simulink library "MBDS_Subsystems"  (R2018b)
settings: Solver=ode45  StartTime=0.0  StopTime=10.0  RelTol=1e-3
undefined symbols (not defined in the file or in its folder): nbo_False, nbo_True
libraries: KIBES_Signal x1438, MBDS_Modules x44, simulink x2
(part 1 of 15)
Description:
  | MBDS project library for Subsystem models
settings Model: Creator=uid60719  LastModifiedBy=uie79669
settings DataIOCC: LimitDataPoints=on  SaveFormat=Array  SignalLoggingSaveFormat=ModelDataLogs
settings OptimizationCC: BlockReduction=off  BooleanDataType=off  ExpressionDepthLimit=2147483647  LifeSpan=inf
settings DebuggingCC: SaveWithParameterizedLinksMsg=none  UnderspecifiedInitializationDetection=Classic  MergeDetectMultiDrivingBlocksExec=none  SignalResolutionControl=TryResolveAllWithWarning  MultiTaskCondExecSysMsg=none  FcnCallInpInsideContextMsg=warning  AllowSymbolicDim=off  StateNameClashWarn=warning  SFUnexpectedBacktrackingDiag=warning  SFNoUnconditionalDefaultTransitionDiag=warning  SFExecutionAtInitializationDiag=none
settings HardwareCC: ProdBitPerPointer=32  ProdBitPerSizeT=32  ProdBitPerPtrDiffT=32  ProdLargestAtomicFloat=None  ProdIntDivRoundTo=Undefined  ProdEndianess=Unspecified  ProdWordSize=32  ProdHWDeviceType=32-bit Generic  TargetUnknown=on
settings ModelReferenceCC: PropagateSignalLabelsOutOfModel=off
settings SFSimCC: SimUseLocalCustomCode=off
settings RTWCC: RTWUseLocalCustomCode=off
settings CodeAppCC: StateflowObjectComments=on
settings GRTTargetCC: TargetLangStandard=C89/C90 (ANSI)  GeneratePreprocessorConditionals=Disable all  CombineOutputUpdateFcns=off  GRTInterface=on
settings ConfigComp: CovMetricSettings=dw  CovHtmlReporting=on  CovSaveCumulativeToWorkspaceVar=on  CovSaveSingleToWorkspaceVar=on  CovExternalEMLEnable=off  CovSFcnEnable=off

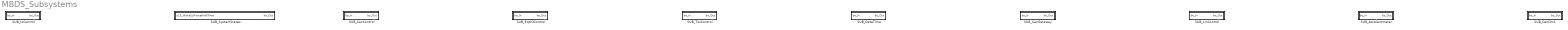
== system MBDS_Subsystems ==
  SUB_Accelerometer : Subsystem  Description=Controls accelerometer signals  mask(SUB_Accelerometer){MBDS_ElementType=Subsystem, MBDS_WorkStatus=In Work, MBDS_LastModified=2023-02-23-17:58:48}
      mask prompts: MBDS_ElementType "MBDS element type:"; MBDS_WorkStatus "Work status:"; MBDS_LastModified "Last modified:"
      mask help: Controls accelerometer signals
      mask Help: eval(['open([workdir(''help_dir:''),''\MBDS_ProjectLibrary.html''])'])
      mask Display: disp('V 1.3')
  SUB_CanControl : Subsystem  Description=CAN Control  mask(SUB_CanControl){MBDS_ElementType=Subsystem, MBDS_WorkStatus=In Work, MBDS_LastModified=2023-02-23-17:58:52}
      mask prompts: MBDS_ElementType "MBDS element type:"; MBDS_WorkStatus "Work status:"; MBDS_LastModified "Last modified:"
      mask help: CAN Control
      mask Help: eval(['open([workdir(''help_dir:''),''\MBDS_ProjectLibrary.html''])'])
      mask Display: disp('V 1.16')
  SUB_CanDm1 : Subsystem  Description=Check DM1 Rx/Tx  mask(SUB_CanDm1){MBDS_ElementType=Subsystem, MBDS_WorkStatus=In Work, MBDS_LastModified=2023-02-23-17:58:48}
      mask prompts: MBDS_ElementType "MBDS element type:"; MBDS_WorkStatus "Work status:"; MBDS_LastModified "Last modified:"
      mask help: Check DM1 Rx/Tx
      mask Help: eval(['open([workdir(''help_dir:''),''\MBDS_ProjectLibrary.html''])'])
      mask Display: disp('V 1.11')
  SUB_CanGateway : Subsystem  Description=CAN Gateways.  mask(SUB_CanGateway){MBDS_ElementType=Subsystem, MBDS_WorkStatus=In Work, MBDS_LastModified=2023-02-23-17:58:50}
      mask prompts: MBDS_ElementType "MBDS element type:"; MBDS_WorkStatus "Work status:"; MBDS_LastModified "Last modified:"
      mask help: CAN Gateways.
      mask Help: eval(['open([workdir(''help_dir:''),''\MBDS_ProjectLibrary.html''])'])
      mask Display: disp('V 1.6')
  SUB_DateTime : Subsystem  Description=Date and Time Control  mask(SUB_DateTime){MBDS_ElementType=Subsystem, MBDS_WorkStatus=In Work, MBDS_LastModified=2023-02-23-17:58:50}
      mask prompts: MBDS_ElementType "MBDS element type:"; MBDS_WorkStatus "Work status:"; MBDS_LastModified "Last modified:"
      mask help: Date and Time Control
      mask Help: eval(['open([workdir(''help_dir:''),''\MBDS_ProjectLibrary.html''])'])
      mask Display: disp('V 1.7')
  SUB_ExpIOControl : Subsystem  Description=Expansion Input/Output Control  mask(SUB_ExpIOControl){MBDS_ElementType=Subsystem, MBDS_WorkStatus=In Work, MBDS_LastModified=2023-02-23-17:58:54}
      mask prompts: MBDS_ElementType "MBDS element type:"; MBDS_WorkStatus "Work status:"; MBDS_LastModified "Last modified:"
      mask help: Expansion Input/Output Control
      mask Help: eval(['open([workdir(''help_dir:''),''\MBDS_ProjectLibrary.html''])'])
      mask Display: disp('V 1.101')
  SUB_IoControl : Subsystem  Description=Input/Output Control  mask(SUB_IoControl){MBDS_ElementType=Subsystem, MBDS_WorkStatus=In Work, MBDS_LastModified=2023-02-23-17:58:58}
      mask prompts: MBDS_ElementType "MBDS element type:"; MBDS_WorkStatus "Work status:"; MBDS_LastModified "Last modified:"
      mask help: Input/Output Control
      mask Help: eval(['open([workdir(''help_dir:''),''\MBDS_ProjectLibrary.html''])'])
      mask Display: disp('V 1.107')
  SUB_LinControl : Subsystem  Description=LIN Control  mask(SUB_LinControl){MBDS_ElementType=Subsystem, MBDS_WorkStatus=In Work, MBDS_LastModified=2023-02-23-17:58:49}
      mask prompts: MBDS_ElementType "MBDS element type:"; MBDS_WorkStatus "Work status:"; MBDS_LastModified "Last modified:"
      mask help: LIN Control
      mask Help: eval(['open([workdir(''help_dir:''),''\MBDS_ProjectLibrary.html''])'])
      mask Display: disp('V 1.27')
  SUB_SystemStates : Subsystem  Description=System States  mask(SUB_SystemStates){MBDS_ElementType=Subsystem, MBDS_WorkStatus=In Work, MBDS_LastModified=2023-02-23-17:58:59}
      mask prompts: MBDS_ElementType "MBDS element type:"; MBDS_WorkStatus "Work status:"; MBDS_LastModified "Last modified:"
      mask help: System States
      mask Help: eval(['open([workdir(''help_dir:''),''\MBDS_ProjectLibrary.html''])'])
      mask Display: disp('V 1.17')
  SUB_TsuControl : Subsystem  Description=TSU Control  mask(SUB_TsuControl){MBDS_ElementType=Subsystem, MBDS_WorkStatus=In Work, MBDS_LastModified=2023-02-23-17:58:51}
      mask prompts: MBDS_ElementType "MBDS element type:"; MBDS_WorkStatus "Work status:"; MBDS_LastModified "Last modified:"
      mask help: TSU Control
      mask Help: eval(['open([workdir(''help_dir:''),''\MBDS_ProjectLibrary.html''])'])
      mask Display: disp('V 1.4')

== system MBDS_Subsystems/SUB_Accelerometer ==
  bo_In : Inport  OutDataTypeStr=boolean
  Constant : Constant  InitFcn=|  Value=true  OutDataTypeStr=boolean
      | if(exist('MBDS_BlockCallback', 'file'))
      |    MBDS_BlockCallback('Update', gcb);  
      | end
  Data Type Conversion : DataTypeConversion  InitFcn=|
      | try
      |    MBDS_BlockCallback('Update', gcb);
      | end
      settings: AttributesFormatString=Saturate: %<SaturateOnIntegerOverflow>
  Data Type Conversion1 : DataTypeConversion  InitFcn=|
      | try
      |    MBDS_BlockCallback('Update', gcb);
      | end
      settings: AttributesFormatString=Saturate: %<SaturateOnIntegerOverflow>
  Data Type Conversion2 : DataTypeConversion  InitFcn=|
      | try
      |    MBDS_BlockCallback('Update', gcb);
      | end
      settings: AttributesFormatString=Saturate: %<SaturateOnIntegerOverflow>
  Ground : Ground  InitFcn=|
      | try
      |    MBDS_BlockCallback('Update', gcb);
      | end
      settings: MoveFcn=UpdateBlockSize(gcb);
  Terminator : Terminator
      settings: MoveFcn=UpdateBlockSize(gcb);
      settings: InitFcn=|
      | try
      |    MBDS_BlockCallback('Update', gcb);
      | end
  in_INOUT_RAMDevice.boSystemWake : KIBES_Signal/KIBES_Signal  MBDS_LibraryBlock=on  DatabaseKey=3  SignalName=INOUT_RAMDevice.boSystemWake  SymbolName=INOUT_RAMDevice_boSystemWake_000003  DataType=boolean  Init=0  Slope=1  Bias=0  DataSize=1  fpDataType=boolean  BlockIOType=Inport  DeviceType=0
  in_IN_InertianSensor.Accelerometer.Ax : KIBES_Signal/KIBES_Signal  MBDS_LibraryBlock=on  DatabaseKey=2138  SignalName=IN_InertianSensor.Accelerometer.Ax  SymbolName=IN_InertianSensor_Accelerometer_Ax_002138  DataType=int16  Init=0  Slope=1  Bias=0  DataSize=1  fpDataType=int16  BlockIOType=Inport  DeviceType=0
  in_IN_InertianSensor.Accelerometer.Ay : KIBES_Signal/KIBES_Signal  MBDS_LibraryBlock=on  DatabaseKey=2137  SignalName=IN_InertianSensor.Accelerometer.Ay  SymbolName=IN_InertianSensor_Accelerometer_Ay_002137  DataType=int16  Init=0  Slope=1  Bias=0  DataSize=1  fpDataType=int16  BlockIOType=Inport  DeviceType=0
  in_IN_InertianSensor.Accelerometer.Az : KIBES_Signal/KIBES_Signal  MBDS_LibraryBlock=on  DatabaseKey=2136  SignalName=IN_InertianSensor.Accelerometer.Az  SymbolName=IN_InertianSensor_Accelerometer_Az_002136  DataType=int16  Init=0  Slope=1  Bias=0  DataSize=1  fpDataType=int16  BlockIOType=Inport  DeviceType=0
  out_OUT_InertianSensor.Accelerometer.DeviceEnable : KIBES_Signal/KIBES_Signal  MBDS_LibraryBlock=on  DatabaseKey=2135  SignalName=OUT_InertianSensor.Accelerometer.DeviceEnable  SymbolName=OUT_InertianSensor_Accelerometer_DeviceEnable_002135  DataType=boolean  Init=0  Slope=1  Bias=0  DataSize=1  fpDataType=boolean  BlockIOType=Outport  DeviceType=0
  out_OUT_PCAN.Tx_Acc.ACCELEROMETER.MessageEnable : KIBES_Signal/KIBES_Signal  MBDS_LibraryBlock=on  DatabaseKey=2134  SignalName=OUT_PCAN.Tx_Acc.ACCELEROMETER.MessageEnable  SymbolName=OUT_PCAN_Tx_Acc_ACCELEROMETER_MessageEnable_002134  DataType=boolean  Init=0  Slope=1  Bias=0  DataSize=1  fpDataType=boolean  BlockIOType=Outport  DeviceType=0
  out_OUT_PCAN.Tx_Acc.ACCELEROMETER.X : KIBES_Signal/KIBES_Signal  MBDS_LibraryBlock=on  DatabaseKey=2131  SignalName=OUT_PCAN.Tx_Acc.ACCELEROMETER.X  SymbolName=OUT_PCAN_Tx_Acc_ACCELEROMETER_X_002131  DataType=uint16  Init=0  Slope=1  Bias=0  DataSize=1  fpDataType=uint16  BlockIOType=Outport  DeviceType=0
  out_OUT_PCAN.Tx_Acc.ACCELEROMETER.Y : KIBES_Signal/KIBES_Signal  MBDS_LibraryBlock=on  DatabaseKey=2132  SignalName=OUT_PCAN.Tx_Acc.ACCELEROMETER.Y  SymbolName=OUT_PCAN_Tx_Acc_ACCELEROMETER_Y_002132  DataType=uint16  Init=0  Slope=1  Bias=0  DataSize=1  fpDataType=uint16  BlockIOType=Outport  DeviceType=0
  out_OUT_PCAN.Tx_Acc.ACCELEROMETER.Z : KIBES_Signal/KIBES_Signal  MBDS_LibraryBlock=on  DatabaseKey=2133  SignalName=OUT_PCAN.Tx_Acc.ACCELEROMETER.Z  SymbolName=OUT_PCAN_Tx_Acc_ACCELEROMETER_Z_002133  DataType=uint16  Init=0  Slope=1  Bias=0  DataSize=1  fpDataType=uint16  BlockIOType=Outport  DeviceType=0
  bo_Out : Outport  OutDataTypeStr=boolean
  wires:
  Data Type Conversion2/1 -> out_OUT_PCAN.Tx_Acc.ACCELEROMETER.Z/1
  Data Type Conversion1/1 -> out_OUT_PCAN.Tx_Acc.ACCELEROMETER.Y/1
  Data Type Conversion/1 -> out_OUT_PCAN.Tx_Acc.ACCELEROMETER.X/1
  in_IN_InertianSensor.Accelerometer.Az/1 -> Data Type Conversion2/1
  in_IN_InertianSensor.Accelerometer.Ay/1 -> Data Type Conversion1/1
  in_IN_InertianSensor.Accelerometer.Ax/1 -> Data Type Conversion/1
  Constant/1 -> out_OUT_InertianSensor.Accelerometer.DeviceEnable/1
  in_INOUT_RAMDevice.boSystemWake/1 -> out_OUT_PCAN.Tx_Acc.ACCELEROMETER.MessageEnable/1
  Ground/1 -> bo_Out/1  "bo_Out"
  bo_In/1 -> Terminator/1

== system MBDS_Subsystems/SUB_CanControl ==
  note: Enable Message Forwarding
  note: SleepMode(0)
      | ShutdownMode(1)
      | ASWFailureMode(2)
      | ModeOverVoltage(3)
      | ModeUnderVoltage(4)
      | LCWakeupSequence(5)
      | TimeoutFailureMode(6)
      |  ActiveMode(7)
      |  SYFlashingMode(8)
  bo_In : Inport  OutDataTypeStr=boolean
  Constant : Constant  InitFcn=|  Value=true  OutDataTypeStr=boolean
      | if(exist('MBDS_BlockCallback', 'file'))
      |    MBDS_BlockCallback('Update', gcb);  
      | end
  Ground : Ground  InitFcn=|
      | try
      |    MBDS_BlockCallback('Update', gcb);
      | end
      settings: MoveFcn=UpdateBlockSize(gcb);
  Terminator : Terminator
      settings: MoveFcn=UpdateBlockSize(gcb);
      settings: InitFcn=|
      | try
      |    MBDS_BlockCallback('Update', gcb);
      | end
  WakeUpSequency : Stateflow chart  TreatAsAtomicUnit=on
      settings: CopyFcn=|
      | if(exist('MBDS_BlockCallback', 'file'))
      |    MBDS_BlockCallback('Copy', gcb);
      | end
  in_IN_DigitalInputs.IN_DIG_36 : KIBES_Signal/KIBES_Signal  MBDS_LibraryBlock=on  DatabaseKey=60  SignalName=IN_DigitalInputs.IN_DIG_36  SymbolName=IN_DigitalInputs_IN_DIG_36_000060  DataType=boolean  Init=0  Slope=1  Bias=0  DataSize=1  fpDataType=boolean  BlockIOType=Inport  DeviceType=0
  out_OUT_ACAN.MessageForwardingEnable : KIBES_Signal/KIBES_Signal  MBDS_LibraryBlock=on  DatabaseKey=2356  SignalName=OUT_ACAN.MessageForwardingEnable  SymbolName=OUT_ACAN_MessageForwardingEnable_002356  DataType=boolean  Init=0  Slope=1  Bias=0  DataSize=1  fpDataType=boolean  BlockIOType=Outport  DeviceType=0
  out_OUT_DCAN.MessageForwardingEnable : KIBES_Signal/KIBES_Signal  MBDS_LibraryBlock=on  DatabaseKey=1337  SignalName=OUT_DCAN.MessageForwardingEnable  SymbolName=OUT_DCAN_MessageForwardingEnable_001337  DataType=boolean  Init=0  Slope=1  Bias=0  DataSize=1  fpDataType=boolean  BlockIOType=Outport  DeviceType=0
  out_OUT_DRCAN.MessageForwardingEnable : KIBES_Signal/KIBES_Signal  MBDS_LibraryBlock=on  DatabaseKey=1335  SignalName=OUT_DRCAN.MessageForwardingEnable  SymbolName=OUT_DRCAN_MessageForwardingEnable_001335  DataType=boolean  Init=0  Slope=1  Bias=0  DataSize=1  fpDataType=boolean  BlockIOType=Outport  DeviceType=0
  out_OUT_FMSCAN.MessageForwardingEnable : KIBES_Signal/KIBES_Signal  MBDS_LibraryBlock=on  DatabaseKey=1336  SignalName=OUT_FMSCAN.MessageForwardingEnable  SymbolName=OUT_FMSCAN_MessageForwardingEnable_001336  DataType=boolean  Init=0  Slope=1  Bias=0  DataSize=1  fpDataType=boolean  BlockIOType=Outport  DeviceType=0
  out_OUT_HCAN.MessageForwardingEnable : KIBES_Signal/KIBES_Signal  MBDS_LibraryBlock=on  DatabaseKey=1340  SignalName=OUT_HCAN.MessageForwardingEnable  SymbolName=OUT_HCAN_MessageForwardingEnable_001340  DataType=boolean  Init=0  Slope=1  Bias=0  DataSize=1  fpDataType=boolean  BlockIOType=Outport  DeviceType=0
  out_OUT_ICAN.BSG_TX_18DA1721.Ctrl50_FcnDA1.MessageEnable : KIBES_Signal/KIBES_Signal  MBDS_LibraryBlock=on  DatabaseKey=2793  SignalName=OUT_ICAN.BSG_TX_18DA1721.Ctrl50_FcnDA1.MessageEnable  SymbolName=OUT_ICAN_BSG_TX_18DA1721_Ctrl50_FcnDA1_MessageEnable_002793  DataType=boolean  Init=0  Slope=1  Bias=0  DataSize=1  fpDataType=boolean  BlockIOType=Outport  DeviceType=0
  out_OUT_ICAN.BSG_TX_18DA1721.Ctrl50_FcnDA2.MessageEnable : KIBES_Signal/KIBES_Signal  MBDS_LibraryBlock=on  DatabaseKey=2795  SignalName=OUT_ICAN.BSG_TX_18DA1721.Ctrl50_FcnDA2.MessageEnable  SymbolName=OUT_ICAN_BSG_TX_18DA1721_Ctrl50_FcnDA2_MessageEnable_002795  DataType=boolean  Init=0  Slope=1  Bias=0  DataSize=1  fpDataType=boolean  BlockIOType=Outport  DeviceType=0
  out_OUT_ICAN.BSG_TX_18DA1721.Ctrl50_ScrDA1.MessageEnable : KIBES_Signal/KIBES_Signal  MBDS_LibraryBlock=on  DatabaseKey=2796  SignalName=OUT_ICAN.BSG_TX_18DA1721.Ctrl50_ScrDA1.MessageEnable  SymbolName=OUT_ICAN_BSG_TX_18DA1721_Ctrl50_ScrDA1_MessageEnable_002796  DataType=boolean  Init=0  Slope=1  Bias=0  DataSize=1  fpDataType=boolean  BlockIOType=Outport  DeviceType=0
  out_OUT_ICAN.BSG_TX_18DA1721.Ctrl50_ScrDA2.MessageEnable : KIBES_Signal/KIBES_Signal  MBDS_LibraryBlock=on  DatabaseKey=2797  SignalName=OUT_ICAN.BSG_TX_18DA1721.Ctrl50_ScrDA2.MessageEnable  SymbolName=OUT_ICAN_BSG_TX_18DA1721_Ctrl50_ScrDA2_MessageEnable_002797  DataType=boolean  Init=0  Slope=1  Bias=0  DataSize=1  fpDataType=boolean  BlockIOType=Outport  DeviceType=0
  out_OUT_ICAN.BSG_TX_18DA1721.Ctrl50_SubView.MessageEnable : KIBES_Signal/KIBES_Signal  MBDS_LibraryBlock=on  DatabaseKey=2794  SignalName=OUT_ICAN.BSG_TX_18DA1721.Ctrl50_SubView.MessageEnable  SymbolName=OUT_ICAN_BSG_TX_18DA1721_Ctrl50_SubView_MessageEnable_002794  DataType=boolean  Init=0  Slope=1  Bias=0  DataSize=1  fpDataType=boolean  BlockIOType=Outport  DeviceType=0
  out_OUT_ICAN.BSG_TX_18DA1721.ICHMI1CTRL.MessageEnable : KIBES_Signal/KIBES_Signal  MBDS_LibraryBlock=on  DatabaseKey=2798  SignalName=OUT_ICAN.BSG_TX_18DA1721.ICHMI1CTRL.MessageEnable  SymbolName=OUT_ICAN_BSG_TX_18DA1721_ICHMI1CTRL_MessageEnable_002798  DataType=boolean  Init=0  Slope=1  Bias=0  DataSize=1  fpDataType=boolean  BlockIOType=Outport  DeviceType=0
  out_OUT_ICAN.BSG_TX_18DA1721.ICOM1CTRL.ICOMCtrl : KIBES_Signal/KIBES_Signal  MBDS_LibraryBlock=on  DatabaseKey=2704  SignalName=OUT_ICAN.BSG_TX_18DA1721.ICOM1CTRL.ICOMCtrl  SymbolName=OUT_ICAN_BSG_TX_18DA1721_ICOM1CTRL_ICOMCtrl_002704  DataType=uint8  Init=1  Slope=1  Bias=0  DataSize=1  fpDataType=uint8  BlockIOType=Outport  DeviceType=0
  out_OUT_ICAN.BSG_TX_18DA1721.ICOM1CTRL.MessageEnable : KIBES_Signal/KIBES_Signal  MBDS_LibraryBlock=on  DatabaseKey=2792  SignalName=OUT_ICAN.BSG_TX_18DA1721.ICOM1CTRL.MessageEnable  SymbolName=OUT_ICAN_BSG_TX_18DA1721_ICOM1CTRL_MessageEnable_002792  DataType=boolean  Init=0  Slope=1  Bias=0  DataSize=1  fpDataType=boolean  BlockIOType=Outport  DeviceType=0
  out_OUT_ICAN.MessageForwardingEnable : KIBES_Signal/KIBES_Signal  MBDS_LibraryBlock=on  DatabaseKey=1342  SignalName=OUT_ICAN.MessageForwardingEnable  SymbolName=OUT_ICAN_MessageForwardingEnable_001342  DataType=boolean  Init=0  Slope=1  Bias=0  DataSize=1  fpDataType=boolean  BlockIOType=Outport  DeviceType=0
  out_OUT_PCAN.MessageForwardingEnable : KIBES_Signal/KIBES_Signal  MBDS_LibraryBlock=on  DatabaseKey=1347  SignalName=OUT_PCAN.MessageForwardingEnable  SymbolName=OUT_PCAN_MessageForwardingEnable_001347  DataType=boolean  Init=0  Slope=1  Bias=0  DataSize=1  fpDataType=boolean  BlockIOType=Outport  DeviceType=0
  bo_Out : Outport  OutDataTypeStr=boolean
  wires:
  in_IN_DigitalInputs.IN_DIG_36/1 -> WakeUpSequency/1(bo_TRM15)
  WakeUpSequency/1(u8_IControlsts) -> out_OUT_ICAN.BSG_TX_18DA1721.ICOM1CTRL.ICOMCtrl/1
  Constant/1 -> out_OUT_DCAN.MessageForwardingEnable/1, out_OUT_DRCAN.MessageForwardingEnable/1, out_OUT_FMSCAN.MessageForwardingEnable/1, out_OUT_HCAN.MessageForwardingEnable/1, out_OUT_ICAN.MessageForwardingEnable/1, out_OUT_PCAN.MessageForwardingEnable/1, out_OUT_ACAN.MessageForwardingEnable/1, out_OUT_ICAN.BSG_TX_18DA1721.Ctrl50_ScrDA2.MessageEnable/1, out_OUT_ICAN.BSG_TX_18DA1721.Ctrl50_FcnDA1.MessageEnable/1, out_OUT_ICAN.BSG_TX_18DA1721.Ctrl50_FcnDA2.MessageEnable/1, out_OUT_ICAN.BSG_TX_18DA1721.Ctrl50_ScrDA1.MessageEnable/1, out_OUT_ICAN.BSG_TX_18DA1721.Ctrl50_SubView.MessageEnable/1, out_OUT_ICAN.BSG_TX_18DA1721.ICHMI1CTRL.MessageEnable/1, out_OUT_ICAN.BSG_TX_18DA1721.ICOM1CTRL.MessageEnable/1
  Ground/1 -> bo_Out/1  "bo_Out"
  bo_In/1 -> Terminator/1

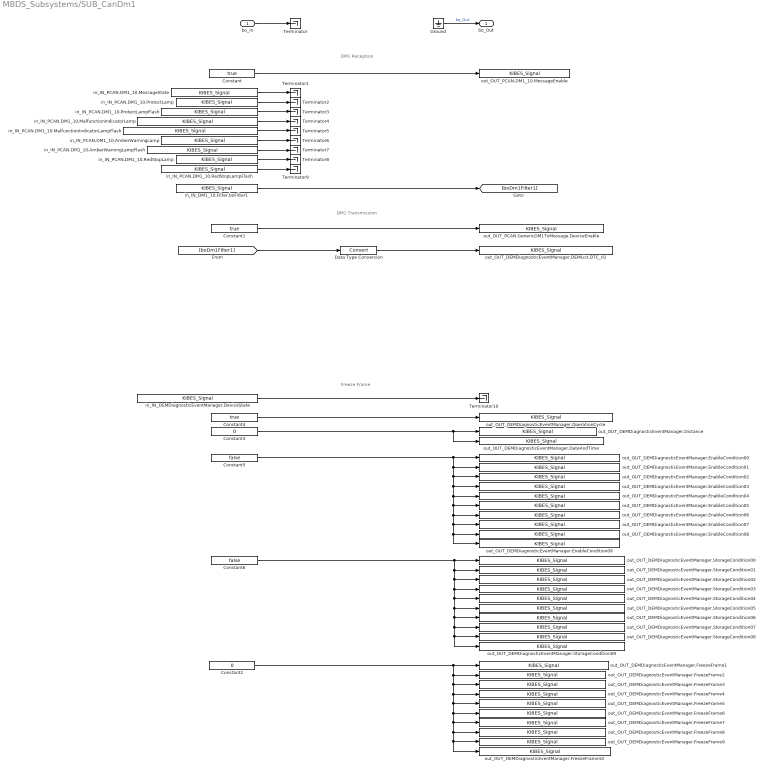
== system MBDS_Subsystems/SUB_CanDm1 ==
  note: Freeze Frame
  note: DM1 Transmission
  note: DM1 Reception
  bo_In : Inport  OutDataTypeStr=boolean
  Constant : Constant  InitFcn=|  Value=true  OutDataTypeStr=boolean
      | if(exist('MBDS_BlockCallback', 'file'))
      |    MBDS_BlockCallback('Update', gcb);  
      | end
  Constant1 : Constant  InitFcn=|  Value=true  OutDataTypeStr=boolean
      | if(exist('MBDS_BlockCallback', 'file'))
      |    MBDS_BlockCallback('Update', gcb);  
      | end
  Constant2 : Constant  InitFcn=|  Value=0  OutDataTypeStr=uint16
      | if(exist('MBDS_BlockCallback', 'file'))
      |    MBDS_BlockCallback('Update', gcb);  
      | end
  Constant3 : Constant  InitFcn=|  Value=0  OutDataTypeStr=uint32
      | if(exist('MBDS_BlockCallback', 'file'))
      |    MBDS_BlockCallback('Update', gcb);  
      | end
  Constant4 : Constant  InitFcn=|  Value=true  OutDataTypeStr=boolean
      | if(exist('MBDS_BlockCallback', 'file'))
      |    MBDS_BlockCallback('Update', gcb);  
      | end
  Constant5 : Constant  InitFcn=|  Value=false  OutDataTypeStr=boolean
      | if(exist('MBDS_BlockCallback', 'file'))
      |    MBDS_BlockCallback('Update', gcb);  
      | end
  Constant6 : Constant  InitFcn=|  Value=false  OutDataTypeStr=boolean
      | if(exist('MBDS_BlockCallback', 'file'))
      |    MBDS_BlockCallback('Update', gcb);  
      | end
  Data Type Conversion : DataTypeConversion  InitFcn=|
      | try
      |    MBDS_BlockCallback('Update', gcb);
      | end
      settings: AttributesFormatString=Saturate: %<SaturateOnIntegerOverflow>
  Ground : Ground  InitFcn=|
      | try
      |    MBDS_BlockCallback('Update', gcb);
      | end
      settings: MoveFcn=UpdateBlockSize(gcb);
  Terminator{,1..10} (11 alike) : Terminator
      settings: MoveFcn=UpdateBlockSize(gcb);
      settings: InitFcn=|
      | try
      |    MBDS_BlockCallback('Update', gcb);
      | end
  in_IN_DEMDiagnosticEventManager.DeviceState : KIBES_Signal/KIBES_Signal  MBDS_LibraryBlock=on  DatabaseKey=2238  SignalName=IN_DEMDiagnosticEventManager.DeviceState  SymbolName=IN_DEMDiagnosticEventManager_DeviceState_002238  DataType=uint16  Init=0  Slope=1  Bias=0  DataSize=1  fpDataType=uint16  BlockIOType=Inport  DeviceType=0
  in_IN_DM1_10.Filter.boFilter1 : KIBES_Signal/KIBES_Signal  MBDS_LibraryBlock=on  DatabaseKey=2234  SignalName=IN_DM1_10.Filter.boFilter1  SymbolName=IN_DM1_10_Filter_boFilter1_002234  DataType=boolean  Init=0  Slope=1  Bias=0  DataSize=1  fpDataType=boolean  BlockIOType=Inport  DeviceType=0
  in_IN_PCAN.DM1_10.AmberWarningLamp : KIBES_Signal/KIBES_Signal  MBDS_LibraryBlock=on  DatabaseKey=2233  SignalName=IN_PCAN.DM1_10.AmberWarningLamp  SymbolName=IN_PCAN_DM1_10_AmberWarningLamp_002233  DataType=boolean  Init=0  Slope=1  Bias=0  DataSize=1  fpDataType=boolean  BlockIOType=Inport  DeviceType=0
  in_IN_PCAN.DM1_10.AmberWarningLampFlash : KIBES_Signal/KIBES_Signal  MBDS_LibraryBlock=on  DatabaseKey=2232  SignalName=IN_PCAN.DM1_10.AmberWarningLampFlash  SymbolName=IN_PCAN_DM1_10_AmberWarningLampFlash_002232  DataType=uint8  Init=0  Slope=1  Bias=0  DataSize=1  fpDataType=uint8  BlockIOType=Inport  DeviceType=0
  in_IN_PCAN.DM1_10.MalfunctionIndicatorLamp : KIBES_Signal/KIBES_Signal  MBDS_LibraryBlock=on  DatabaseKey=2231  SignalName=IN_PCAN.DM1_10.MalfunctionIndicatorLamp  SymbolName=IN_PCAN_DM1_10_MalfunctionIndicatorLamp_002231  DataType=boolean  Init=0  Slope=1  Bias=0  DataSize=1  fpDataType=boolean  BlockIOType=Inport  DeviceType=0
  in_IN_PCAN.DM1_10.MalfunctionIndicatorLampFlash : KIBES_Signal/KIBES_Signal  MBDS_LibraryBlock=on  DatabaseKey=2230  SignalName=IN_PCAN.DM1_10.MalfunctionIndicatorLampFlash  SymbolName=IN_PCAN_DM1_10_MalfunctionIndicatorLampFlash_002230  DataType=uint8  Init=0  Slope=1  Bias=0  DataSize=1  fpDataType=uint8  BlockIOType=Inport  DeviceType=0
  in_IN_PCAN.DM1_10.MessageState : KIBES_Signal/KIBES_Signal  MBDS_LibraryBlock=on  DatabaseKey=2228  SignalName=IN_PCAN.DM1_10.MessageState  SymbolName=IN_PCAN_DM1_10_MessageState_002228  DataType=uint16  Init=0  Slope=1  Bias=0  DataSize=1  fpDataType=uint16  BlockIOType=Inport  DeviceType=0
  in_IN_PCAN.DM1_10.ProtectLamp : KIBES_Signal/KIBES_Signal  MBDS_LibraryBlock=on  DatabaseKey=2227  SignalName=IN_PCAN.DM1_10.ProtectLamp  SymbolName=IN_PCAN_DM1_10_ProtectLamp_002227  DataType=boolean  Init=0  Slope=1  Bias=0  DataSize=1  fpDataType=boolean  BlockIOType=Inport  DeviceType=0
  in_IN_PCAN.DM1_10.ProtectLampFlash : KIBES_Signal/KIBES_Signal  MBDS_LibraryBlock=on  DatabaseKey=2226  SignalName=IN_PCAN.DM1_10.ProtectLampFlash  SymbolName=IN_PCAN_DM1_10_ProtectLampFlash_002226  DataType=uint8  Init=0  Slope=1  Bias=0  DataSize=1  fpDataType=uint8  BlockIOType=Inport  DeviceType=0
  in_IN_PCAN.DM1_10.RedStopLamp : KIBES_Signal/KIBES_Signal  MBDS_LibraryBlock=on  DatabaseKey=2225  SignalName=IN_PCAN.DM1_10.RedStopLamp  SymbolName=IN_PCAN_DM1_10_RedStopLamp_002225  DataType=boolean  Init=0  Slope=1  Bias=0  DataSize=1  fpDataType=boolean  BlockIOType=Inport  DeviceType=0
  in_IN_PCAN.DM1_10.RedStopLampFlash : KIBES_Signal/KIBES_Signal  MBDS_LibraryBlock=on  DatabaseKey=2224  SignalName=IN_PCAN.DM1_10.RedStopLampFlash  SymbolName=IN_PCAN_DM1_10_RedStopLampFlash_002224  DataType=uint8  Init=0  Slope=1  Bias=0  DataSize=1  fpDataType=uint8  BlockIOType=Inport  DeviceType=0
  out_OUT_DEMDiagnosticEventManager.DEMList.DTC_01 : KIBES_Signal/KIBES_Signal  MBDS_LibraryBlock=on  DatabaseKey=2237  SignalName=OUT_DEMDiagnosticEventManager.DEMList.DTC_01  SymbolName=OUT_DEMDiagnosticEventManager_DEMList_DTC_01_002237  DataType=uint8  Init=0  Slope=1  Bias=0  DataSize=1  fpDataType=uint8  BlockIOType=Outport  DeviceType=0
  out_OUT_DEMDiagnosticEventManager.DateAndTime : KIBES_Signal/KIBES_Signal  MBDS_LibraryBlock=on  DatabaseKey=2242  SignalName=OUT_DEMDiagnosticEventManager.DateAndTime  SymbolName=OUT_DEMDiagnosticEventManager_DateAndTime_002242  DataType=uint32  Init=0  Slope=1  Bias=0  DataSize=1  fpDataType=uint32  BlockIOType=Outport  DeviceType=0
  out_OUT_DEMDiagnosticEventManager.Distance : KIBES_Signal/KIBES_Signal  MBDS_LibraryBlock=on  DatabaseKey=2243  SignalName=OUT_DEMDiagnosticEventManager.Distance  SymbolName=OUT_DEMDiagnosticEventManager_Distance_002243  DataType=uint32  Init=0  Slope=1  Bias=0  DataSize=1  fpDataType=uint32  BlockIOType=Outport  DeviceType=0
  out_OUT_DEMDiagnosticEventManager.EnableCondition00 : KIBES_Signal/KIBES_Signal  MBDS_LibraryBlock=on  DatabaseKey=2239  SignalName=OUT_DEMDiagnosticEventManager.EnableCondition00  SymbolName=OUT_DEMDiagnosticEventManager_EnableCondition00_002239  DataType=boolean  Init=0  Slope=1  Bias=0  DataSize=1  fpDataType=boolean  BlockIOType=Outport  DeviceType=0
  out_OUT_DEMDiagnosticEventManager.EnableCondition01 : KIBES_Signal/KIBES_Signal  MBDS_LibraryBlock=on  DatabaseKey=2245  SignalName=OUT_DEMDiagnosticEventManager.EnableCondition01  SymbolName=OUT_DEMDiagnosticEventManager_EnableCondition01_002245  DataType=boolean  Init=0  Slope=1  Bias=0  DataSize=1  fpDataType=boolean  BlockIOType=Outport  DeviceType=0
  out_OUT_DEMDiagnosticEventManager.EnableCondition02 : KIBES_Signal/KIBES_Signal  MBDS_LibraryBlock=on  DatabaseKey=2246  SignalName=OUT_DEMDiagnosticEventManager.EnableCondition02  SymbolName=OUT_DEMDiagnosticEventManager_EnableCondition02_002246  DataType=boolean  Init=0  Slope=1  Bias=0  DataSize=1  fpDataType=boolean  BlockIOType=Outport  DeviceType=0
  out_OUT_DEMDiagnosticEventManager.EnableCondition03 : KIBES_Signal/KIBES_Signal  MBDS_LibraryBlock=on  DatabaseKey=2247  SignalName=OUT_DEMDiagnosticEventManager.EnableCondition03  SymbolName=OUT_DEMDiagnosticEventManager_EnableCondition03_002247  DataType=boolean  Init=0  Slope=1  Bias=0  DataSize=1  fpDataType=boolean  BlockIOType=Outport  DeviceType=0
  out_OUT_DEMDiagnosticEventManager.EnableCondition04 : KIBES_Signal/KIBES_Signal  MBDS_LibraryBlock=on  DatabaseKey=2248  SignalName=OUT_DEMDiagnosticEventManager.EnableCondition04  SymbolName=OUT_DEMDiagnosticEventManager_EnableCondition04_002248  DataType=boolean  Init=0  Slope=1  Bias=0  DataSize=1  fpDataType=boolean  BlockIOType=Outport  DeviceType=0
  out_OUT_DEMDiagnosticEventManager.EnableCondition05 : KIBES_Signal/KIBES_Signal  MBDS_LibraryBlock=on  DatabaseKey=2249  SignalName=OUT_DEMDiagnosticEventManager.EnableCondition05  SymbolName=OUT_DEMDiagnosticEventManager_EnableCondition05_002249  DataType=boolean  Init=0  Slope=1  Bias=0  DataSize=1  fpDataType=boolean  BlockIOType=Outport  DeviceType=0
  out_OUT_DEMDiagnosticEventManager.EnableCondition06 : KIBES_Signal/KIBES_Signal  MBDS_LibraryBlock=on  DatabaseKey=2250  SignalName=OUT_DEMDiagnosticEventManager.EnableCondition06  SymbolName=OUT_DEMDiagnosticEventManager_EnableCondition06_002250  DataType=boolean  Init=0  Slope=1  Bias=0  DataSize=1  fpDataType=boolean  BlockIOType=Outport  DeviceType=0
  out_OUT_DEMDiagnosticEventManager.EnableCondition07 : KIBES_Signal/KIBES_Signal  MBDS_LibraryBlock=on  DatabaseKey=2251  SignalName=OUT_DEMDiagnosticEventManager.EnableCondition07  SymbolName=OUT_DEMDiagnosticEventManager_EnableCondition07_002251  DataType=boolean  Init=0  Slope=1  Bias=0  DataSize=1  fpDataType=boolean  BlockIOType=Outport  DeviceType=0
  out_OUT_DEMDiagnosticEventManager.EnableCondition08 : KIBES_Signal/KIBES_Signal  MBDS_LibraryBlock=on  DatabaseKey=2252  SignalName=OUT_DEMDiagnosticEventManager.EnableCondition08  SymbolName=OUT_DEMDiagnosticEventManager_EnableCondition08_002252  DataType=boolean  Init=0  Slope=1  Bias=0  DataSize=1  fpDataType=boolean  BlockIOType=Outport  DeviceType=0
  out_OUT_DEMDiagnosticEventManager.EnableCondition09 : KIBES_Signal/KIBES_Signal  MBDS_LibraryBlock=on  DatabaseKey=2244  SignalName=OUT_DEMDiagnosticEventManager.EnableCondition09  SymbolName=OUT_DEMDiagnosticEventManager_EnableCondition09_002244  DataType=boolean  Init=0  Slope=1  Bias=0  DataSize=1  fpDataType=boolean  BlockIOType=Outport  DeviceType=0
  out_OUT_DEMDiagnosticEventManager.FreezeFrame1 : KIBES_Signal/KIBES_Signal  MBDS_LibraryBlock=on  DatabaseKey=2241  SignalName=OUT_DEMDiagnosticEventManager.FreezeFrame1  SymbolName=OUT_DEMDiagnosticEventManager_FreezeFrame1_002241  DataType=uint16  Init=0  Slope=1  Bias=0  DataSize=1  fpDataType=uint16  BlockIOType=Outport  DeviceType=0
  out_OUT_DEMDiagnosticEventManager.FreezeFrame10 : KIBES_Signal/KIBES_Signal  MBDS_LibraryBlock=on  DatabaseKey=2270  SignalName=OUT_DEMDiagnosticEventManager.FreezeFrame10  SymbolName=OUT_DEMDiagnosticEventManager_FreezeFrame10_002270  DataType=uint16  Init=0  Slope=1  Bias=0  DataSize=1  fpDataType=uint16  BlockIOType=Outport  DeviceType=0
  out_OUT_DEMDiagnosticEventManager.FreezeFrame2 : KIBES_Signal/KIBES_Signal  MBDS_LibraryBlock=on  DatabaseKey=2253  SignalName=OUT_DEMDiagnosticEventManager.FreezeFrame2  SymbolName=OUT_DEMDiagnosticEventManager_FreezeFrame2_002253  DataType=uint16  Init=0  Slope=1  Bias=0  DataSize=1  fpDataType=uint16  BlockIOType=Outport  DeviceType=0
  out_OUT_DEMDiagnosticEventManager.FreezeFrame3 : KIBES_Signal/KIBES_Signal  MBDS_LibraryBlock=on  DatabaseKey=2254  SignalName=OUT_DEMDiagnosticEventManager.FreezeFrame3  SymbolName=OUT_DEMDiagnosticEventManager_FreezeFrame3_002254  DataType=uint16  Init=0  Slope=1  Bias=0  DataSize=1  fpDataType=uint16  BlockIOType=Outport  DeviceType=0
  out_OUT_DEMDiagnosticEventManager.FreezeFrame4 : KIBES_Signal/KIBES_Signal  MBDS_LibraryBlock=on  DatabaseKey=2255  SignalName=OUT_DEMDiagnosticEventManager.FreezeFrame4  SymbolName=OUT_DEMDiagnosticEventManager_FreezeFrame4_002255  DataType=uint16  Init=0  Slope=1  Bias=0  DataSize=1  fpDataType=uint16  BlockIOType=Outport  DeviceType=0
  out_OUT_DEMDiagnosticEventManager.FreezeFrame5 : KIBES_Signal/KIBES_Signal  MBDS_LibraryBlock=on  DatabaseKey=2256  SignalName=OUT_DEMDiagnosticEventManager.FreezeFrame5  SymbolName=OUT_DEMDiagnosticEventManager_FreezeFrame5_002256  DataType=uint16  Init=0  Slope=1  Bias=0  DataSize=1  fpDataType=uint16  BlockIOType=Outport  DeviceType=0
  out_OUT_DEMDiagnosticEventManager.FreezeFrame6 : KIBES_Signal/KIBES_Signal  MBDS_LibraryBlock=on  DatabaseKey=2266  SignalName=OUT_DEMDiagnosticEventManager.FreezeFrame6  SymbolName=OUT_DEMDiagnosticEventManager_FreezeFrame6_002266  DataType=uint16  Init=0  Slope=1  Bias=0  DataSize=1  fpDataType=uint16  BlockIOType=Outport  DeviceType=0
  out_OUT_DEMDiagnosticEventManager.FreezeFrame7 : KIBES_Signal/KIBES_Signal  MBDS_LibraryBlock=on  DatabaseKey=2267  SignalName=OUT_DEMDiagnosticEventManager.FreezeFrame7  SymbolName=OUT_DEMDiagnosticEventManager_FreezeFrame7_002267  DataType=uint16  Init=0  Slope=1  Bias=0  DataSize=1  fpDataType=uint16  BlockIOType=Outport  DeviceType=0
  out_OUT_DEMDiagnosticEventManager.FreezeFrame8 : KIBES_Signal/KIBES_Signal  MBDS_LibraryBlock=on  DatabaseKey=2268  SignalName=OUT_DEMDiagnosticEventManager.FreezeFrame8  SymbolName=OUT_DEMDiagnosticEventManager_FreezeFrame8_002268  DataType=uint16  Init=0  Slope=1  Bias=0  DataSize=1  fpDataType=uint16  BlockIOType=Outport  DeviceType=0
  out_OUT_DEMDiagnosticEventManager.FreezeFrame9 : KIBES_Signal/KIBES_Signal  MBDS_LibraryBlock=on  DatabaseKey=2269  SignalName=OUT_DEMDiagnosticEventManager.FreezeFrame9  SymbolName=OUT_DEMDiagnosticEventManager_FreezeFrame9_002269  DataType=uint16  Init=0  Slope=1  Bias=0  DataSize=1  fpDataType=uint16  BlockIOType=Outport  DeviceType=0
  out_OUT_DEMDiagnosticEventManager.OperationCycle : KIBES_Signal/KIBES_Signal  MBDS_LibraryBlock=on  DatabaseKey=2235  SignalName=OUT_DEMDiagnosticEventManager.OperationCycle  SymbolName=OUT_DEMDiagnosticEventManager_OperationCycle_002235  DataType=boolean  Init=0  Slope=1  Bias=0  DataSize=1  fpDataType=boolean  BlockIOType=Outport  DeviceType=0
  out_OUT_DEMDiagnosticEventManager.StorageCondition00 : KIBES_Signal/KIBES_Signal  MBDS_LibraryBlock=on  DatabaseKey=2240  SignalName=OUT_DEMDiagnosticEventManager.StorageCondition00  SymbolName=OUT_DEMDiagnosticEventManager_StorageCondition00_002240  DataType=boolean  Init=0  Slope=1  Bias=0  DataSize=1  fpDataType=boolean  BlockIOType=Outport  DeviceType=0
  out_OUT_DEMDiagnosticEventManager.StorageCondition01 : KIBES_Signal/KIBES_Signal  MBDS_LibraryBlock=on  DatabaseKey=2258  SignalName=OUT_DEMDiagnosticEventManager.StorageCondition01  SymbolName=OUT_DEMDiagnosticEventManager_StorageCondition01_002258  DataType=boolean  Init=0  Slope=1  Bias=0  DataSize=1  fpDataType=boolean  BlockIOType=Outport  DeviceType=0
  out_OUT_DEMDiagnosticEventManager.StorageCondition02 : KIBES_Signal/KIBES_Signal  MBDS_LibraryBlock=on  DatabaseKey=2259  SignalName=OUT_DEMDiagnosticEventManager.StorageCondition02  SymbolName=OUT_DEMDiagnosticEventManager_StorageCondition02_002259  DataType=boolean  Init=0  Slope=1  Bias=0  DataSize=1  fpDataType=boolean  BlockIOType=Outport  DeviceType=0
  out_OUT_DEMDiagnosticEventManager.StorageCondition03 : KIBES_Signal/KIBES_Signal  MBDS_LibraryBlock=on  DatabaseKey=2260  SignalName=OUT_DEMDiagnosticEventManager.StorageCondition03  SymbolName=OUT_DEMDiagnosticEventManager_StorageCondition03_002260  DataType=boolean  Init=0  Slope=1  Bias=0  DataSize=1  fpDataType=boolean  BlockIOType=Outport  DeviceType=0
  out_OUT_DEMDiagnosticEventManager.StorageCondition04 : KIBES_Signal/KIBES_Signal  MBDS_LibraryBlock=on  DatabaseKey=2261  SignalName=OUT_DEMDiagnosticEventManager.StorageCondition04  SymbolName=OUT_DEMDiagnosticEventManager_StorageCondition04_002261  DataType=boolean  Init=0  Slope=1  Bias=0  DataSize=1  fpDataType=boolean  BlockIOType=Outport  DeviceType=0
  out_OUT_DEMDiagnosticEventManager.StorageCondition05 : KIBES_Signal/KIBES_Signal  MBDS_LibraryBlock=on  DatabaseKey=2262  SignalName=OUT_DEMDiagnosticEventManager.StorageCondition05  SymbolName=OUT_DEMDiagnosticEventManager_StorageCondition05_002262  DataType=boolean  Init=0  Slope=1  Bias=0  DataSize=1  fpDataType=boolean  BlockIOType=Outport  DeviceType=0
  out_OUT_DEMDiagnosticEventManager.StorageCondition06 : KIBES_Signal/KIBES_Signal  MBDS_LibraryBlock=on  DatabaseKey=2263  SignalName=OUT_DEMDiagnosticEventManager.StorageCondition06  SymbolName=OUT_DEMDiagnosticEventManager_StorageCondition06_002263  DataType=boolean  Init=0  Slope=1  Bias=0  DataSize=1  fpDataType=boolean  BlockIOType=Outport  DeviceType=0
  out_OUT_DEMDiagnosticEventManager.StorageCondition07 : KIBES_Signal/KIBES_Signal  MBDS_LibraryBlock=on  DatabaseKey=2264  SignalName=OUT_DEMDiagnosticEventManager.StorageCondition07  SymbolName=OUT_DEMDiagnosticEventManager_StorageCondition07_002264  DataType=boolean  Init=0  Slope=1  Bias=0  DataSize=1  fpDataType=boolean  BlockIOType=Outport  DeviceType=0
  out_OUT_DEMDiagnosticEventManager.StorageCondition08 : KIBES_Signal/KIBES_Signal  MBDS_LibraryBlock=on  DatabaseKey=2265  SignalName=OUT_DEMDiagnosticEventManager.StorageCondition08  SymbolName=OUT_DEMDiagnosticEventManager_StorageCondition08_002265  DataType=boolean  Init=0  Slope=1  Bias=0  DataSize=1  fpDataType=boolean  BlockIOType=Outport  DeviceType=0
  out_OUT_DEMDiagnosticEventManager.StorageCondition09 : KIBES_Signal/KIBES_Signal  MBDS_LibraryBlock=on  DatabaseKey=2257  SignalName=OUT_DEMDiagnosticEventManager.StorageCondition09  SymbolName=OUT_DEMDiagnosticEventManager_StorageCondition09_002257  DataType=boolean  Init=0  Slope=1  Bias=0  DataSize=1  fpDataType=boolean  BlockIOType=Outport  DeviceType=0
  out_OUT_PCAN.DM1_10.MessageEnable : KIBES_Signal/KIBES_Signal  MBDS_LibraryBlock=on  DatabaseKey=2229  SignalName=OUT_PCAN.DM1_10.MessageEnable  SymbolName=OUT_PCAN_DM1_10_MessageEnable_002229  DataType=boolean  Init=0  Slope=1  Bias=0  DataSize=1  fpDataType=boolean  BlockIOType=Outport  DeviceType=0
  out_OUT_PCAN.GenericDM1TxMessage.DeviceEnable : KIBES_Signal/KIBES_Signal  MBDS_LibraryBlock=on  DatabaseKey=2236  SignalName=OUT_PCAN.GenericDM1TxMessage.DeviceEnable  SymbolName=OUT_PCAN_GenericDM1TxMessage_DeviceEnable_002236  DataType=boolean  Init=0  Slope=1  Bias=0  DataSize=1  fpDataType=boolean  BlockIOType=Outport  DeviceType=0
  bo_Out : Outport  OutDataTypeStr=boolean
  wires:
  Constant6/1 -> out_OUT_DEMDiagnosticEventManager.StorageCondition00/1, out_OUT_DEMDiagnosticEventManager.StorageCondition01/1, out_OUT_DEMDiagnosticEventManager.StorageCondition02/1, out_OUT_DEMDiagnosticEventManager.StorageCondition03/1, out_OUT_DEMDiagnosticEventManager.StorageCondition04/1, out_OUT_DEMDiagnosticEventManager.StorageCondition05/1, out_OUT_DEMDiagnosticEventManager.StorageCondition06/1, out_OUT_DEMDiagnosticEventManager.StorageCondition07/1, out_OUT_DEMDiagnosticEventManager.StorageCondition08/1, out_OUT_DEMDiagnosticEventManager.StorageCondition09/1
  Constant5/1 -> out_OUT_DEMDiagnosticEventManager.EnableCondition00/1, out_OUT_DEMDiagnosticEventManager.EnableCondition01/1, out_OUT_DEMDiagnosticEventManager.EnableCondition02/1, out_OUT_DEMDiagnosticEventManager.EnableCondition03/1, out_OUT_DEMDiagnosticEventManager.EnableCondition04/1, out_OUT_DEMDiagnosticEventManager.EnableCondition05/1, out_OUT_DEMDiagnosticEventManager.EnableCondition06/1, out_OUT_DEMDiagnosticEventManager.EnableCondition07/1, out_OUT_DEMDiagnosticEventManager.EnableCondition08/1, out_OUT_DEMDiagnosticEventManager.EnableCondition09/1
  Constant4/1 -> out_OUT_DEMDiagnosticEventManager.OperationCycle/1
  Constant3/1 -> out_OUT_DEMDiagnosticEventManager.Distance/1, out_OUT_DEMDiagnosticEventManager.DateAndTime/1
  Constant2/1 -> out_OUT_DEMDiagnosticEventManager.FreezeFrame1/1, out_OUT_DEMDiagnosticEventManager.FreezeFrame2/1, out_OUT_DEMDiagnosticEventManager.FreezeFrame3/1, out_OUT_DEMDiagnosticEventManager.FreezeFrame4/1, out_OUT_DEMDiagnosticEventManager.FreezeFrame5/1, out_OUT_DEMDiagnosticEventManager.FreezeFrame6/1, out_OUT_DEMDiagnosticEventManager.FreezeFrame7/1, out_OUT_DEMDiagnosticEventManager.FreezeFrame8/1, out_OUT_DEMDiagnosticEventManager.FreezeFrame9/1, out_OUT_DEMDiagnosticEventManager.FreezeFrame10/1
  in_IN_DEMDiagnosticEventManager.DeviceState/1 -> Terminator10/1
  Data Type Conversion/1 -> out_OUT_DEMDiagnosticEventManager.DEMList.DTC_01/1
  [boDm1Filter1] -> Data Type Conversion/1
  Constant1/1 -> out_OUT_PCAN.GenericDM1TxMessage.DeviceEnable/1
  in_IN_DM1_10.Filter.boFilter1/1 -> [boDm1Filter1]
  in_IN_PCAN.DM1_10.RedStopLampFlash/1 -> Terminator9/1
  in_IN_PCAN.DM1_10.RedStopLamp/1 -> Terminator8/1
  in_IN_PCAN.DM1_10.AmberWarningLampFlash/1 -> Terminator7/1
  in_IN_PCAN.DM1_10.AmberWarningLamp/1 -> Terminator6/1
  in_IN_PCAN.DM1_10.MalfunctionIndicatorLampFlash/1 -> Terminator5/1
  in_IN_PCAN.DM1_10.MalfunctionIndicatorLamp/1 -> Terminator4/1
  in_IN_PCAN.DM1_10.ProtectLampFlash/1 -> Terminator3/1
  in_IN_PCAN.DM1_10.ProtectLamp/1 -> Terminator2/1
  in_IN_PCAN.DM1_10.MessageState/1 -> Terminator1/1
  Constant/1 -> out_OUT_PCAN.DM1_10.MessageEnable/1
  Ground/1 -> bo_Out/1  "bo_Out"
  bo_In/1 -> Terminator/1

== system MBDS_Subsystems/SUB_CanGateway ==
  note: A-CAN Gateway
  note: P-CAN Gateway
  note: I-CAN Gateway
  note: H-CAN Gateway
  note: FMS-CAN Gateway
  note: DR-CAN Gateway
  note: D-CAN Gateway
  bo_In : Inport  OutDataTypeStr=boolean
  Constant : Constant  InitFcn=|  Value=true  OutDataTypeStr=boolean
      | if(exist('MBDS_BlockCallback', 'file'))
      |    MBDS_BlockCallback('Update', gcb);  
      | end
  Constant1 : Constant  InitFcn=|  Value=true  OutDataTypeStr=boolean
      | if(exist('MBDS_BlockCallback', 'file'))
      |    MBDS_BlockCallback('Update', gcb);  
      | end
  Constant2 : Constant  InitFcn=|  Value=true  OutDataTypeStr=boolean
      | if(exist('MBDS_BlockCallback', 'file'))
      |    MBDS_BlockCallback('Update', gcb);  
      | end
  Constant3 : Constant  InitFcn=|  Value=true  OutDataTypeStr=boolean
      | if(exist('MBDS_BlockCallback', 'file'))
      |    MBDS_BlockCallback('Update', gcb);  
      | end
  Constant4 : Constant  InitFcn=|  Value=true  OutDataTypeStr=boolean
      | if(exist('MBDS_BlockCallback', 'file'))
      |    MBDS_BlockCallback('Update', gcb);  
      | end
  Constant5 : Constant  InitFcn=|  Value=true  OutDataTypeStr=boolean
      | if(exist('MBDS_BlockCallback', 'file'))
      |    MBDS_BlockCallback('Update', gcb);  
      | end
  Constant6 : Constant  InitFcn=|  Value=true  OutDataTypeStr=boolean
      | if(exist('MBDS_BlockCallback', 'file'))
      |    MBDS_BlockCallback('Update', gcb);  
      | end
  Ground : Ground  InitFcn=|
      | try
      |    MBDS_BlockCallback('Update', gcb);
      | end
      settings: MoveFcn=UpdateBlockSize(gcb);
  Terminator : Terminator
      settings: MoveFcn=UpdateBlockSize(gcb);
      settings: InitFcn=|
      | try
      |    MBDS_BlockCallback('Update', gcb);
      | end
  out_OUT_ACAN.GW_18DAF1E1.MessageEnable : KIBES_Signal/KIBES_Signal  MBDS_LibraryBlock=on  DatabaseKey=2357  SignalName=OUT_ACAN.GW_18DAF1E1.MessageEnable  SymbolName=OUT_ACAN_GW_18DAF1E1_MessageEnable_002357  DataType=boolean  Init=0  Slope=1  Bias=0  DataSize=1  fpDataType=boolean  BlockIOType=Outport  DeviceType=0
  out_OUT_DCAN.GW_00000501.MessageEnable : KIBES_Signal/KIBES_Signal  MBDS_LibraryBlock=on  DatabaseKey=1327  SignalName=OUT_DCAN.GW_00000501.MessageEnable  SymbolName=OUT_DCAN_GW_00000501_MessageEnable_001327  DataType=boolean  Init=0  Slope=1  Bias=0  DataSize=1  fpDataType=boolean  BlockIOType=Outport  DeviceType=0
  out_OUT_DCAN.GW_00000502.MessageEnable : KIBES_Signal/KIBES_Signal  MBDS_LibraryBlock=on  DatabaseKey=1328  SignalName=OUT_DCAN.GW_00000502.MessageEnable  SymbolName=OUT_DCAN_GW_00000502_MessageEnable_001328  DataType=boolean  Init=0  Slope=1  Bias=0  DataSize=1  fpDataType=boolean  BlockIOType=Outport  DeviceType=0
  out_OUT_DCAN.GW_00000503.MessageEnable : KIBES_Signal/KIBES_Signal  MBDS_LibraryBlock=on  DatabaseKey=1329  SignalName=OUT_DCAN.GW_00000503.MessageEnable  SymbolName=OUT_DCAN_GW_00000503_MessageEnable_001329  DataType=boolean  Init=0  Slope=1  Bias=0  DataSize=1  fpDataType=boolean  BlockIOType=Outport  DeviceType=0
  out_OUT_DCAN.GW_00000504.MessageEnable : KIBES_Signal/KIBES_Signal  MBDS_LibraryBlock=on  DatabaseKey=1330  SignalName=OUT_DCAN.GW_00000504.MessageEnable  SymbolName=OUT_DCAN_GW_00000504_MessageEnable_001330  DataType=boolean  Init=0  Slope=1  Bias=0  DataSize=1  fpDataType=boolean  BlockIOType=Outport  DeviceType=0
  out_OUT_DCAN.GW_00000FF1.MessageEnable : KIBES_Signal/KIBES_Signal  MBDS_LibraryBlock=on  DatabaseKey=1331  SignalName=OUT_DCAN.GW_00000FF1.MessageEnable  SymbolName=OUT_DCAN_GW_00000FF1_MessageEnable_001331  DataType=boolean  Init=0  Slope=1  Bias=0  DataSize=1  fpDataType=boolean  BlockIOType=Outport  DeviceType=0
  out_OUT_DCAN.GW_18DA17F0.MessageEnable : KIBES_Signal/KIBES_Signal  MBDS_LibraryBlock=on  DatabaseKey=1332  SignalName=OUT_DCAN.GW_18DA17F0.MessageEnable  SymbolName=OUT_DCAN_GW_18DA17F0_MessageEnable_001332  DataType=boolean  Init=0  Slope=1  Bias=0  DataSize=1  fpDataType=boolean  BlockIOType=Outport  DeviceType=0
  out_OUT_DCAN.GW_18DA17F1.MessageEnable : KIBES_Signal/KIBES_Signal  MBDS_LibraryBlock=on  DatabaseKey=1333  SignalName=OUT_DCAN.GW_18DA17F1.MessageEnable  SymbolName=OUT_DCAN_GW_18DA17F1_MessageEnable_001333  DataType=boolean  Init=0  Slope=1  Bias=0  DataSize=1  fpDataType=boolean  BlockIOType=Outport  DeviceType=0
  out_OUT_DCAN.GW_18DAE1F1.MessageEnable : KIBES_Signal/KIBES_Signal  MBDS_LibraryBlock=on  DatabaseKey=1334  SignalName=OUT_DCAN.GW_18DAE1F1.MessageEnable  SymbolName=OUT_DCAN_GW_18DAE1F1_MessageEnable_001334  DataType=boolean  Init=0  Slope=1  Bias=0  DataSize=1  fpDataType=boolean  BlockIOType=Outport  DeviceType=0
  out_OUT_DRCAN.GW_00000FF6.MessageEnable : KIBES_Signal/KIBES_Signal  MBDS_LibraryBlock=on  DatabaseKey=1338  SignalName=OUT_DRCAN.GW_00000FF6.MessageEnable  SymbolName=OUT_DRCAN_GW_00000FF6_MessageEnable_001338  DataType=boolean  Init=0  Slope=1  Bias=0  DataSize=1  fpDataType=boolean  BlockIOType=Outport  DeviceType=0
  out_OUT_FMSCAN.GW_00000FF5.MessageEnable : KIBES_Signal/KIBES_Signal  MBDS_LibraryBlock=on  DatabaseKey=1339  SignalName=OUT_FMSCAN.GW_00000FF5.MessageEnable  SymbolName=OUT_FMSCAN_GW_00000FF5_MessageEnable_001339  DataType=boolean  Init=0  Slope=1  Bias=0  DataSize=1  fpDataType=boolean  BlockIOType=Outport  DeviceType=0
  out_OUT_HCAN.GW_00000FF7.MessageEnable : KIBES_Signal/KIBES_Signal  MBDS_LibraryBlock=on  DatabaseKey=1341  SignalName=OUT_HCAN.GW_00000FF7.MessageEnable  SymbolName=OUT_HCAN_GW_00000FF7_MessageEnable_001341  DataType=boolean  Init=0  Slope=1  Bias=0  DataSize=1  fpDataType=boolean  BlockIOType=Outport  DeviceType=0
  out_OUT_ICAN.GW_00000600.MessageEnable : KIBES_Signal/KIBES_Signal  MBDS_LibraryBlock=on  DatabaseKey=1343  SignalName=OUT_ICAN.GW_00000600.MessageEnable  SymbolName=OUT_ICAN_GW_00000600_MessageEnable_001343  DataType=boolean  Init=0  Slope=1  Bias=0  DataSize=1  fpDataType=boolean  BlockIOType=Outport  DeviceType=0
  out_OUT_ICAN.GW_00000FF4.MessageEnable : KIBES_Signal/KIBES_Signal  MBDS_LibraryBlock=on  DatabaseKey=1344  SignalName=OUT_ICAN.GW_00000FF4.MessageEnable  SymbolName=OUT_ICAN_GW_00000FF4_MessageEnable_001344  DataType=boolean  Init=0  Slope=1  Bias=0  DataSize=1  fpDataType=boolean  BlockIOType=Outport  DeviceType=0
  out_OUT_ICAN.GW_18DAF017.MessageEnable : KIBES_Signal/KIBES_Signal  MBDS_LibraryBlock=on  DatabaseKey=1345  SignalName=OUT_ICAN.GW_18DAF017.MessageEnable  SymbolName=OUT_ICAN_GW_18DAF017_MessageEnable_001345  DataType=boolean  Init=0  Slope=1  Bias=0  DataSize=1  fpDataType=boolean  BlockIOType=Outport  DeviceType=0
  out_OUT_ICAN.GW_18DAF117.MessageEnable : KIBES_Signal/KIBES_Signal  MBDS_LibraryBlock=on  DatabaseKey=1346  SignalName=OUT_ICAN.GW_18DAF117.MessageEnable  SymbolName=OUT_ICAN_GW_18DAF117_MessageEnable_001346  DataType=boolean  Init=0  Slope=1  Bias=0  DataSize=1  fpDataType=boolean  BlockIOType=Outport  DeviceType=0
  out_OUT_PCAN.GW_00000FF3.MessageEnable : KIBES_Signal/KIBES_Signal  MBDS_LibraryBlock=on  DatabaseKey=1348  SignalName=OUT_PCAN.GW_00000FF3.MessageEnable  SymbolName=OUT_PCAN_GW_00000FF3_MessageEnable_001348  DataType=boolean  Init=0  Slope=1  Bias=0  DataSize=1  fpDataType=boolean  BlockIOType=Outport  DeviceType=0
  bo_Out : Outport  OutDataTypeStr=boolean
  wires:
  Constant6/1 -> out_OUT_ACAN.GW_18DAF1E1.MessageEnable/1
  Constant5/1 -> out_OUT_ICAN.GW_00000FF4.MessageEnable/1, out_OUT_ICAN.GW_18DAF017.MessageEnable/1, out_OUT_ICAN.GW_18DAF117.MessageEnable/1, out_OUT_PCAN.GW_00000FF3.MessageEnable/1
  Constant4/1 -> out_OUT_ICAN.GW_00000600.MessageEnable/1
  Constant3/1 -> out_OUT_HCAN.GW_00000FF7.MessageEnable/1
  Constant2/1 -> out_OUT_FMSCAN.GW_00000FF5.MessageEnable/1
  Constant1/1 -> out_OUT_DRCAN.GW_00000FF6.MessageEnable/1
  Constant/1 -> out_OUT_DCAN.GW_00000501.MessageEnable/1, out_OUT_DCAN.GW_00000502.MessageEnable/1, out_OUT_DCAN.GW_00000503.MessageEnable/1, out_OUT_DCAN.GW_00000504.MessageEnable/1, out_OUT_DCAN.GW_00000FF1.MessageEnable/1, out_OUT_DCAN.GW_18DAE1F1.MessageEnable/1, out_OUT_DCAN.GW_18DA17F1.MessageEnable/1, out_OUT_DCAN.GW_18DA17F0.MessageEnable/1
  Ground/1 -> bo_Out/1  "bo_Out"
  bo_In/1 -> Terminator/1
